simulink model "LaoWang_Test"  (R2022a)
settings: Solver=VariableStepAuto  StartTime=0.0  StopTime=10.0  RelTol=1e-3
libraries: Solver_SF x1
settings Model: Creator=HaiChen  LastModifiedBy=HaiChen

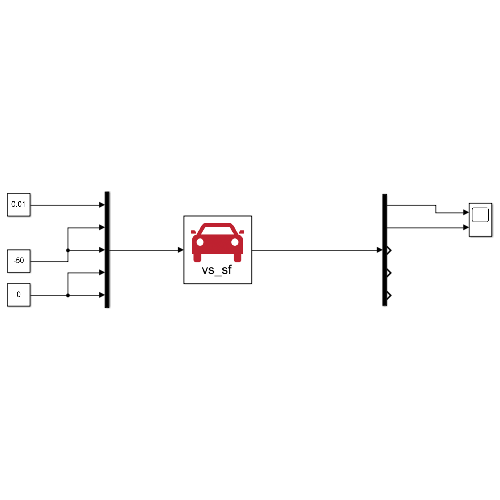
[thumbnail: Simulink's stored preview of the top-level diagram]
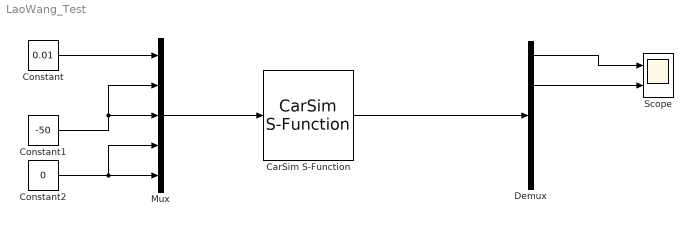
== system LaoWang_Test ==
  CarSim S-Function : Solver_SF/CarSim S-Function  Priority=1  SIMFILE=LaoWang_Test.sim
  Constant : Constant  Value=0.01
  Constant1 : Constant  Value=-50
  Constant2 : Constant  Value=0
  Demux : Demux  Outputs=5
  Mux : Mux  Inputs=5
  Scope : Scope  NumInputPorts=2
  wires:
  Constant/1 -> Mux/1
  Constant1/1 -> Mux/3, Mux/2
  Mux/1 -> CarSim S-Function/1
  CarSim S-Function/1 -> Demux/1
  Demux/1 -> Scope/1
  Demux/2 -> Scope/2
  Constant2/1 -> Mux/5, Mux/4
